simulink model "controller_sketch"  (R2023b)
settings: Solver=VariableStepAuto  StartTime=0.0  StopTime=10  RelTol=1e-3
settings Model: Creator=Andrew Petruska  LastModifiedBy=chris
settings SolverCC: AlgebraicLoopSolver=TrustRegion
settings DebuggingCC: UnconnectedInputMsg=warning  UnconnectedOutputMsg=warning  UnconnectedLineMsg=warning
settings ModelReferenceCC: EnableRefExpFcnMdlSchedulingChecks=on

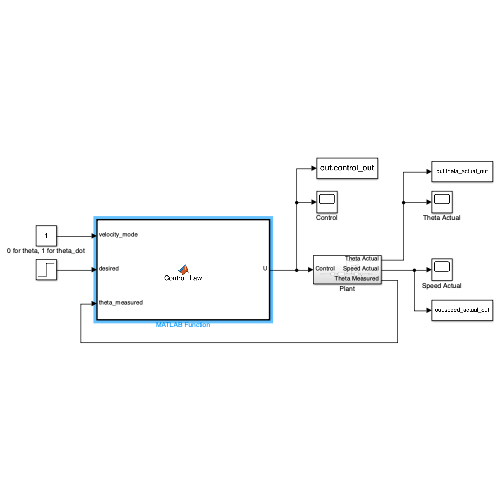
[thumbnail: Simulink's stored preview of the top-level diagram]
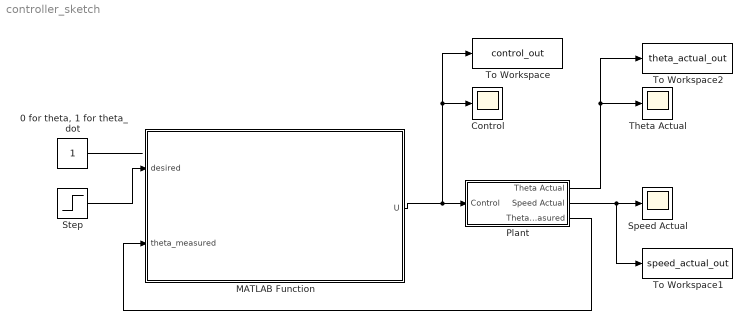
== system controller_sketch ==
  "0 for theta, 1 for theta_dot" : Constant
  Control : Scope
  MATLAB Function : MATLAB Function  TreatAsAtomicUnit=on
  Plant : Subsystem
  Speed Actual : Scope
  Step : Step  After=10  SampleTime=0
  Theta Actual : Scope
  To Workspace : ToWorkspace  VariableName=control_out  SaveFormat=Timeseries  SampleTime=-1
  To Workspace1 : ToWorkspace  VariableName=speed_actual_out  SaveFormat=Timeseries  SampleTime=-1
  To Workspace2 : ToWorkspace  VariableName=theta_actual_out  SaveFormat=Timeseries  SampleTime=-1
  wires:
  Plant/3(Theta Measured) -> MATLAB Function/2(theta_measured)
  MATLAB Function/1(U) -> Plant/1(Control), To Workspace/1, Control/1
  Plant/1(Theta Actual) -> To Workspace2/1, Theta Actual/1
  Plant/2(Speed Actual) -> To Workspace1/1, Speed Actual/1
  Step/1 -> MATLAB Function/1(desired)
  "0 for theta, 1 for theta_dot"/1 -> ?

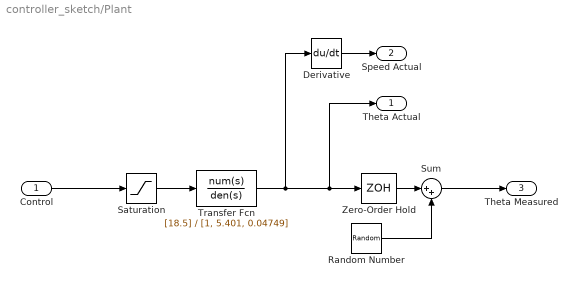
== system controller_sketch/Plant ==
  Control : Inport
  Derivative : Derivative
  Random Number : RandomNumber  Variance=.25^2  SampleTime=0.001
  Saturation : Saturate  UpperLimit=5  LowerLimit=-5
  Sum : Sum  Inputs=|++
  Transfer Fcn : TransferFcn  Numerator=[18.5]  Denominator=[1, 5.401, 0.04749]  ContinuousStateAttributes='Theta'
  Zero-Order Hold : ZeroOrderHold  SampleTime=0.001
  Theta Actual : Outport
  Speed Actual : Outport  Port=2
  Theta Measured : Outport  Port=3
  wires:
  Control/1 -> Saturation/1
  Transfer Fcn/1 -> Derivative/1, Zero-Order Hold/1, Theta Actual/1
  Random Number/1 -> Sum/2
  Sum/1 -> Theta Measured/1
  Saturation/1 -> Transfer Fcn/1
  Zero-Order Hold/1 -> Sum/1
  Derivative/1 -> Speed Actual/1

== matlab function controller_sketch/MATLAB Function ==
  data: U output; desired input; theta_measured input
function U = Control_Law( desired, theta_measured)

persistent Kp A B output_last input_last theta_target dT;

if isempty(A) % Initialize on first call
   Kp = 298.9930; % Kp coeff 
   A = [2.01392719190951,-1.92386890220897]; % A coeff 
   B = [1,-0.909941710299450]; % B coeff
  
   dT = 0.001; % 1kHz update
   output_last = 0; % dont change
   input_last = theta_measured; % dont change
   theta_target = 0; % dont change
end

% Control Law
output_this = (A(1) * theta_measured) + (A(2) * input_last) - (B(2)*output_last);

% Save current to last for next iteration.
output_last = output_this; 
input_last = theta_measured;


theta_target = desired;



U = Kp*(theta_target - output_this); % Final control calculation.
end
